simulink model "Demodulation"  (R2023b)
settings: Solver=VariableStepAuto  StartTime=0.0  StopTime=10.0  RelTol=1e-3
libraries: dspfdesign x1
settings Model: Creator=satyamagrawal  LastModifiedBy=satyamagrawal

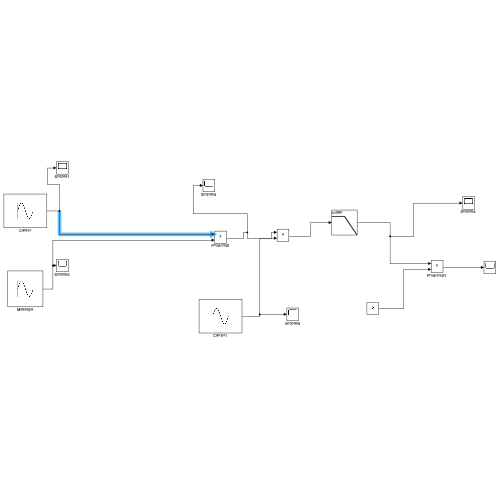
[thumbnail: Simulink's stored preview of the top-level diagram]
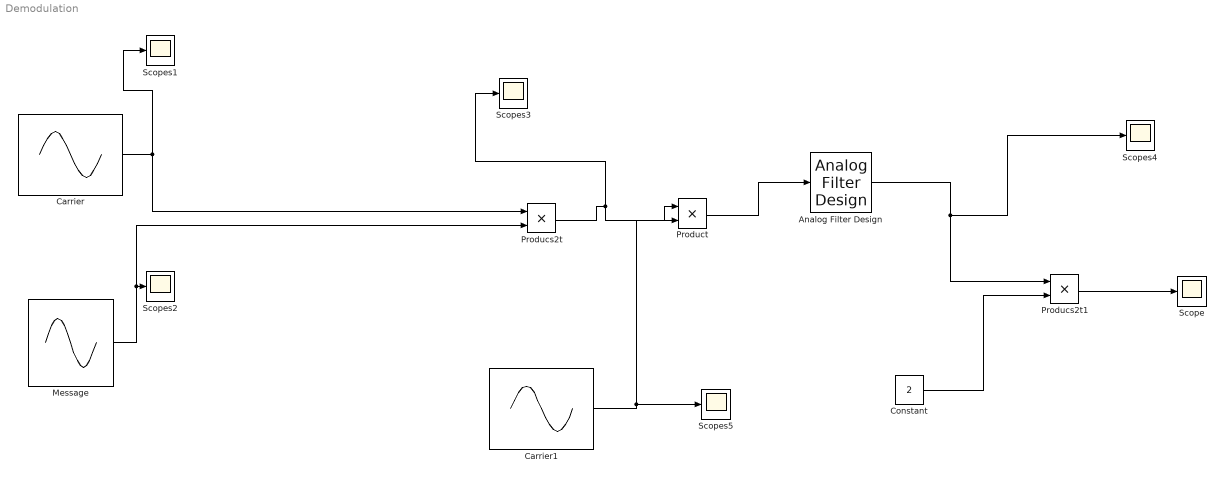
== system Demodulation ==
  Analog Filter Design : dspfdesign/Analog Filter Design  method=Butterworth  filttype=Lowpass  N=8  Wlo=10  Whi=80  Rp=2  Rs=40
  Carrier : Sin  Frequency=10  SampleTime=0
  Carrier1 : Sin  Frequency=10  SampleTime=0
  Constant : Constant  Value=2
  Message : Sin  SampleTime=0
  Producs2t : Product
  Producs2t1 : Product
  Product : Product
  Scope : Scope
  Scopes{1..5} (5 alike) : Scope
  wires:
  Carrier/1 -> Scopes1/1, Producs2t/1
  Message/1 -> Producs2t/2, Scopes2/1
  Carrier1/1 -> Product/2, Scopes5/1
  Producs2t/1 -> Scopes3/1, Product/1
  Product/1 -> Analog Filter Design/1
  Analog Filter Design/1 -> Producs2t1/1, Scopes4/1
  Constant/1 -> Producs2t1/2
  Producs2t1/1 -> Scope/1
